simulink model "Plant_Emulator"  (R2018b)
settings: Solver=VariableStepAuto  StartTime=0.0  StopTime=10.0  RelTol=1e-3
settings Model: Creator=jayakumarav  LastModifiedBy=hiterd
settings DebuggingCC: LibraryContextMissingDiagnostic=none
settings SFSimCC: SimUseLocalCustomCode=off
settings RTWCC: RTWUseLocalCustomCode=off

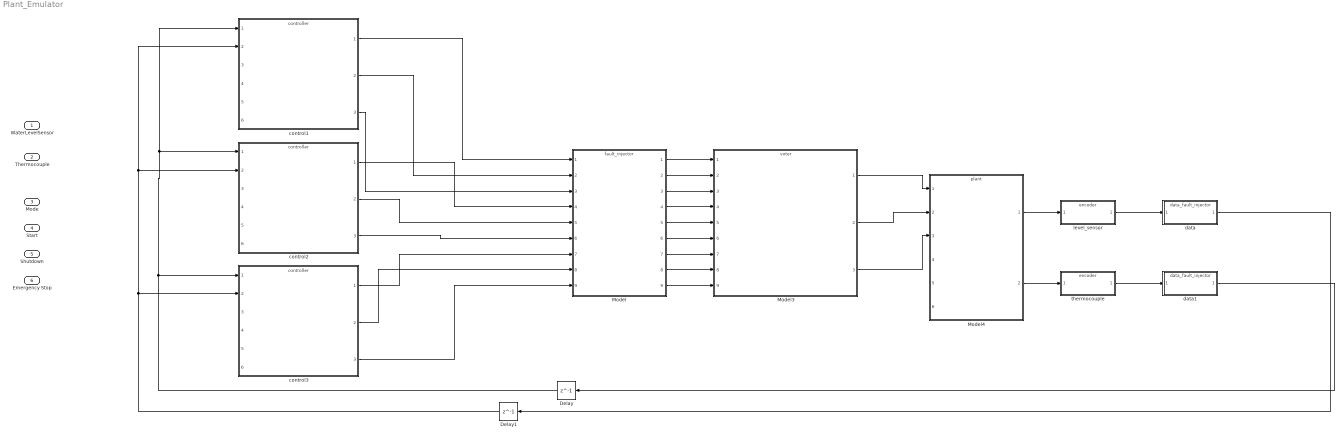
== system Plant_Emulator ==
  WaterLevelSensor : Inport
  Thermocouple : Inport  Port=2
  Mode : Inport  Port=3
  Start : Inport  Port=4
  Shutdown : Inport  Port=5
  Emergency Stop : Inport  Port=6
  Delay : Delay  DelayLength=1  InitialCondition=0
  Delay1 : Delay  DelayLength=1  InitialCondition=0
  Model : ModelReference  ModelNameDialog=fault_injector.slx  SimulationMode=Normal  ModelReferenceVersion=1.25
  Model3 : ModelReference  ModelNameDialog=voter.slx  SimulationMode=Normal  ModelReferenceVersion=1.15
  Model4 : ModelReference  ModelNameDialog=plant.slx  SimulationMode=Normal  ModelReferenceVersion=1.17
  control1 : ModelReference  ModelNameDialog=controller.slx  SimulationMode=Normal  ModelReferenceVersion=1.19
  control2 : ModelReference  ModelNameDialog=controller.slx  SimulationMode=Normal  ModelReferenceVersion=1.19
  control3 : ModelReference  ModelNameDialog=controller.slx  SimulationMode=Normal  ModelReferenceVersion=1.19
  data : ModelReference  ModelNameDialog=data_fault_injector.slx  SimulationMode=Normal  ModelReferenceVersion=1.20
  data1 : ModelReference  ModelNameDialog=data_fault_injector.slx  SimulationMode=Normal  ModelReferenceVersion=1.20
  level_sensor : ModelReference  ModelNameDialog=encoder.slx  SimulationMode=Normal  ModelReferenceVersion=1.20
  thermocouple : ModelReference  ModelNameDialog=encoder.slx  SimulationMode=Normal  ModelReferenceVersion=1.20
  wires:
  control1/3 -> Model/3
  control1/2 -> Model/2
  control1/1 -> Model/1
  control2/2 -> Model/5
  control2/3 -> Model/6
  control2/1 -> Model/4
  Model3/1 -> Model4/1
  Model3/2 -> Model4/2
  Model3/3 -> Model4/3
  thermocouple/1 -> data1/1
  level_sensor/1 -> data/1
  Delay1/1 -> control3/2, control2/2, control1/2
  Delay/1 -> control3/1, control2/1, control1/1
  control3/1 -> Model/7
  control3/2 -> Model/8
  control3/3 -> Model/9
  Model4/1 -> level_sensor/1
  Model4/2 -> thermocouple/1
  Model/1 -> Model3/1
  Model/2 -> Model3/2
  Model/3 -> Model3/3
  Model/4 -> Model3/4
  Model/5 -> Model3/5
  Model/6 -> Model3/6
  Model/7 -> Model3/7
  Model/8 -> Model3/8
  Model/9 -> Model3/9
  data/1 -> Delay1/1
  data1/1 -> Delay/1
